simulink model "lab3_step2"  (R2019b)
settings: Solver=VariableStepAuto  StartTime=0.0  StopTime=stop_time  RelTol=1e-3
InitFcn:
  | %Read in the audio file
  | [input_wav_signal, Fs_in] = audioread('acoustic.wav');
  | % Fs_in = 11025 and we need to convert this to Fs = 48k
  | 
  | % COnvert the Sampling rate to 48 kHz
  | signal = resample(input_wav_signal, 48000, 11025);
  | Fs = 48000; % This is out desired sample rate that we converted to
  | Ts = 1/Fs;    % and the associated sample period.
  | 
  | % Put signal into a timeseries format
  | timevals = [0:length(signal)-1]*Ts;
  | input_signal = timeseries(signal,timevals);
  | 
  | % Set the simulation stop time
  | stop_time = length(signal) * Ts; % set the simulation time the same length as the input signal
  | 
  | 
  | % Fixed-point precision we want the signal converted to.
  | W_bits = 32;
  | F_bits = 28;
StopFcn:
  | y_out = output_signal.Data(:);
  | plot(y_out)
  | soundsc(y_out,Fs)
undefined symbols (not defined in the file): magnitude
settings Model: Creator=yassi  LastModifiedBy=yassi
settings DataIOCC: ReturnWorkspaceOutputs=off

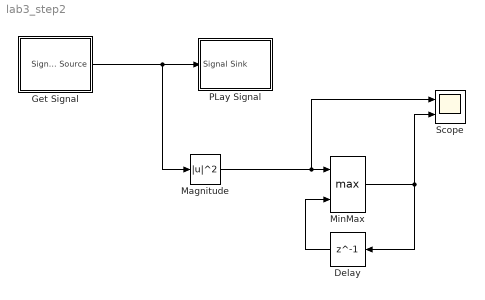
== system lab3_step2 ==
  Delay : Delay  DelayLength=1
  Get Signal : Subsystem
  Magnitude : Math  Operator=magnitude^2  RndMeth=Zero  SaturateOnIntegerOverflow=on
  MinMax : MinMax  Function=max  Inputs=2
  PLay Signal : Subsystem
  Scope : Scope  NumInputPorts=2
  wires:
  Get Signal/1(Signal Source) -> Magnitude/1, PLay Signal/1(Signal Sink)
  Magnitude/1 -> Scope/1, MinMax/1
  MinMax/1 -> Scope/2, Delay/1
  Delay/1 -> MinMax/2

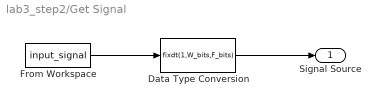
== system lab3_step2/Get Signal ==
  Data Type Conversion : DataTypeConversion  OutDataTypeStr=fixdt(1,W_bits,F_bits)
  From Workspace : FromWorkspace  VariableName=input_signal  SampleTime=Ts
  Signal Source : Outport
  wires:
  From Workspace/1 -> Data Type Conversion/1
  Data Type Conversion/1 -> Signal Source/1

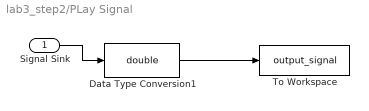
== system lab3_step2/PLay Signal ==
  Signal Sink : Inport
  Data Type Conversion1 : DataTypeConversion  OutDataTypeStr=double
  To Workspace : ToWorkspace  VariableName=output_signal  SaveFormat=Timeseries  SampleTime=-1
  wires:
  Data Type Conversion1/1 -> To Workspace/1
  Signal Sink/1 -> Data Type Conversion1/1
